simulink model "HIL_sim"  (Simulink 7.8)
settings: Solver=FixedStepDiscrete  StartTime=0.0  StopTime=1000  FixedStep=.01  RelTol=1e-3
InitFcn:
  | common
  | Busses
  | physical_constants
values from neighbouring files (symbols this model uses):
  T_step = 0.01    [boat_constants.m]    (also in common.m)
libraries: etargetslib x3, dspnetwork x2, simulink x1, aerolibanimutils x1
settings Model: Creator=Administrator  LastModifiedBy=Bryant  ExtModeAutoUpdateStatusClock=off  BufferReuse=off
settings DataIOCC: MaxDataPoints=1  SaveOutput=off  SignalLogging=off
settings OptimizationCC: BlockReduction=off  InlineParams=on  InlineInvariantSignals=on  BufferReuse=off  InitFltsAndDblsToZero=on  EfficientMapNaN2IntZero=off  LifeSpan=30  SimCompilerOptimization=On
settings DebuggingCC: ReadBeforeWriteMsg=DisableAll  SaveWithParameterizedLinksMsg=none  UnderspecifiedInitializationDetection=Simplified  UniqueDataStoreMsg=error  AssertControl=DisableAll
settings HardwareCC: ProdHWDeviceType=Generic->Unspecified (assume 32-bit Generic)  TargetIntDivRoundTo=Zero  TargetEndianess=LittleEndian  TargetHWDeviceType=Microchip->dsPIC
settings SFSimCC: SimParseCustomCode=off
settings CodeAppCC: MaxIdLength=128

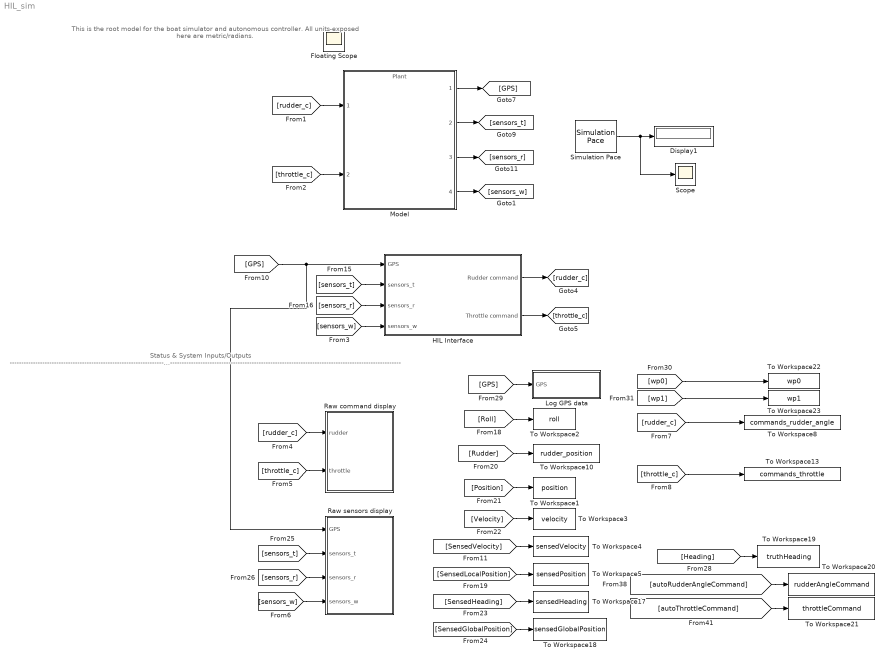
== system HIL_sim ==
  note: This is the root model for the boat simulator and autonomous controller. All
      | units exposed here are metric/radians.
  note: Status & System Inputs/Outputs
      | ---------------------------------------------------------------------------------------------------------------------------------------------------------------------------------------------------------------------------------------------------------
  Display1 : Display
      settings: Decimation=20
  HIL Interface : Subsystem
  Log GPS data : Subsystem
  Model : ModelReference  ModelNameDialog=Plant  SimulationMode=Normal  ModelReferenceVersion=1.14  CopyOfModelName=Plant  DefaultDataLogging=on
  Raw command display : Subsystem
  Raw sensors display : Subsystem
  Scope : Scope
      settings: SaveName=paceError  DataFormat=Array
  Simulation Pace : aerolibanimutils/Simulation Pace  SimulationPace=1  SleepMode=MATLAB Thread  OutputPaceError=on  SampleTime=T_step
      settings: AttributesFormatString=%<SimulationPace> sec/sec
  To Workspace1 : ToWorkspace  VariableName=position  SampleTime=-1  SaveFormat=Array
  To Workspace10 : ToWorkspace  VariableName=rudder_position  SampleTime=-1  SaveFormat=Array
  To Workspace13 : ToWorkspace  VariableName=commands_throttle  SampleTime=-1  SaveFormat=Array
  To Workspace17 : ToWorkspace  VariableName=sensedHeading  SampleTime=-1  SaveFormat=Array
  To Workspace18 : ToWorkspace  VariableName=sensedGlobalPosition  SampleTime=-1  SaveFormat=Array
  To Workspace19 : ToWorkspace  VariableName=truthHeading  SampleTime=-1  SaveFormat=Array
  To Workspace2 : ToWorkspace  VariableName=roll  SampleTime=-1  SaveFormat=Array
  To Workspace20 : ToWorkspace  VariableName=rudderAngleCommand  SampleTime=-1  SaveFormat=Array
  To Workspace21 : ToWorkspace  VariableName=throttleCommand  SampleTime=-1  SaveFormat=Array
  To Workspace22 : ToWorkspace  VariableName=wp0  SampleTime=-1  SaveFormat=Array
  To Workspace23 : ToWorkspace  VariableName=wp1  SampleTime=-1  SaveFormat=Array
  To Workspace3 : ToWorkspace  VariableName=velocity  SampleTime=-1  SaveFormat=Array
  To Workspace4 : ToWorkspace  VariableName=sensedVelocity  SampleTime=-1  SaveFormat=Array
  To Workspace5 : ToWorkspace  VariableName=sensedPosition  SampleTime=-1  SaveFormat=Array
  To Workspace8 : ToWorkspace  VariableName=commands_rudder_angle  SampleTime=-1  SaveFormat=Array
  Floating Scope : Scope
      settings: Floating=on
  wires:
  Model/3 -> [sensors_r]
  [rudder_c] -> Model/1
  [throttle_c] -> Model/2
  Model/1 -> [GPS]
  Model/2 -> [sensors_t]
  HIL Interface/1(Rudder command) -> [rudder_c]
  HIL Interface/2(Throttle command) -> [throttle_c]
  [sensors_r] -> HIL Interface/3(sensors_r)
  [sensors_t] -> HIL Interface/2(sensors_t)
  [GPS] -> HIL Interface/1(GPS), Raw sensors display/1(GPS)
  Model/4 -> [sensors_w]
  [rudder_c] -> Raw command display/1(rudder)
  [throttle_c] -> Raw command display/2(throttle)
  [sensors_t] -> Raw sensors display/2(sensors_t)
  [sensors_r] -> Raw sensors display/3(sensors_r)
  [Roll] -> To Workspace2/1
  [Rudder] -> To Workspace10/1
  [Position] -> To Workspace1/1
  [throttle_c] -> To Workspace13/1
  [rudder_c] -> To Workspace8/1
  [Velocity] -> To Workspace3/1
  [SensedVelocity] -> To Workspace4/1
  [SensedLocalPosition] -> To Workspace5/1
  [SensedHeading] -> To Workspace17/1
  [SensedGlobalPosition] -> To Workspace18/1
  [Heading] -> To Workspace19/1
  [autoRudderAngleCommand] -> To Workspace20/1
  [autoThrottleCommand] -> To Workspace21/1
  [GPS] -> Log GPS data/1(GPS)
  [wp0] -> To Workspace22/1
  [wp1] -> To Workspace23/1
  Simulation Pace/1 -> Display1/1, Scope/1
  [sensors_w] -> HIL Interface/4(sensors_w)
  [sensors_w] -> Raw sensors display/4(sensors_w)

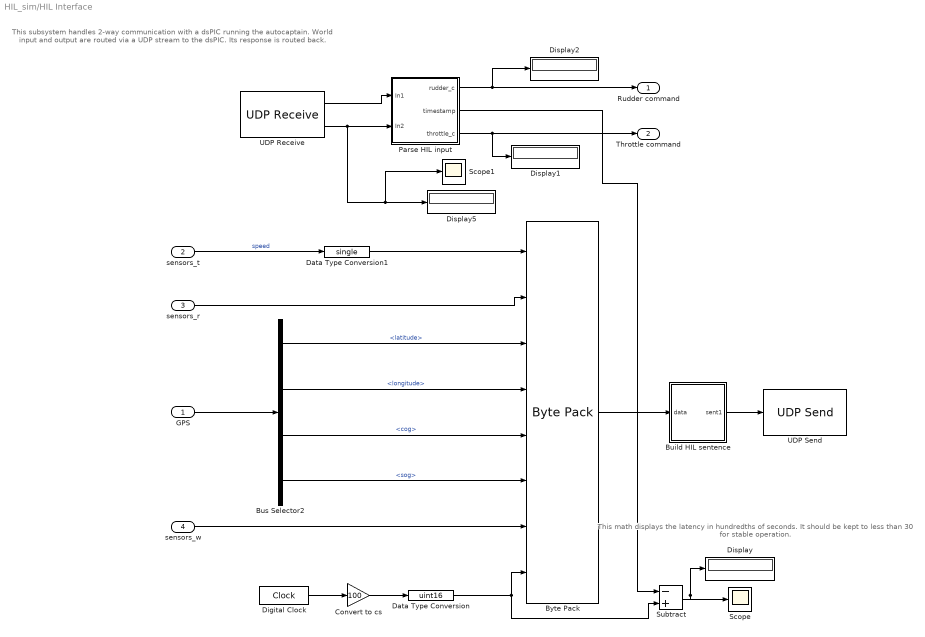
== system HIL_sim/HIL Interface ==
  note: This subsystem handles 2-way communication with a dsPIC running
      | the autocaptain. World input and output are routed via a UDP stream
      | to the dsPIC. Its response is routed back.
  note: This math displays the latency in hundredths of seconds.
      | It should be kept to less than 30 for stable operation.
  GPS : Inport
  sensors_t : Inport  Port=2
  sensors_r : Inport  Port=3
  sensors_w : Inport  Port=4
  Build HIL sentence : Subsystem
  Bus Selector2 : BusSelector  OutputSignals=latitude,longitude,cog,sog
  Byte Pack : etargetslib/Byte Pack  datatypes={'single','single','int32','int32','uint16','uint16','single','uint16'}  byteAlign=1
  Convert to cs : Gain  Gain=100
  Data Type Conversion : DataTypeConversion  OutDataTypeStr=uint16  RndMeth=Simplest
  Data Type Conversion1 : DataTypeConversion  OutDataTypeStr=single  RndMeth=Simplest
  Digital Clock : DigitalClock  SampleTime=.01
  Display{,1..2,5} (4 alike) : Display
  Parse HIL input : Subsystem
  Scope : Scope
      settings: YMin=40  YMax=92.5  SaveName=latency  DataFormat=Array
  Scope1 : Scope
      settings: YMin=40  YMax=92.5  SaveName=latency1  DataFormat=Array
  Subtract : Sum  Inputs=-+  OutDataTypeStr=int16
  UDP Receive : dspnetwork/UDP Receive  localURL='0.0.0.0'  localPort=14551  remoteURL='10.0.0.1'  remotePort=-1  recvBufferSize=44  dims=22  signalDatatype=uint8  isVarSize=off  showBlockingTime=on  blockingTime=0  sampletime=0.01  blockPlatform=HOST
  UDP Send : dspnetwork/UDP Send  remoteURL='10.0.0.1'  remotePort=14550  localURL='255.255.255.255'  localPortSource=Automatically determine  localPort=15000  sampletime=-1  blockPlatform=HOST  separateLengthPort=0
  Rudder command : Outport
  Throttle command : Outport  Port=2
  wires:
  Parse HIL input/1(rudder_c) -> Rudder command/1, Display2/1
  GPS/1 -> Bus Selector2/1
  Parse HIL input/3(throttle_c) -> Throttle command/1, Display1/1
  Byte Pack/1 -> Build HIL sentence/1(data)
  sensors_t/1 -> Data Type Conversion1/1  "speed"
  Build HIL sentence/1(sent1) -> UDP Send/1
  Parse HIL input/2(timestamp) -> Subtract/1
  Convert to cs/1 -> Data Type Conversion/1
  Digital Clock/1 -> Convert to cs/1
  Data Type Conversion/1 -> Subtract/2, Byte Pack/8
  Subtract/1 -> Scope/1, Display/1
  Data Type Conversion1/1 -> Byte Pack/1
  sensors_r/1 -> Byte Pack/2
  Bus Selector2/1 -> Byte Pack/3  "<latitude>"
  Bus Selector2/2 -> Byte Pack/4  "<longitude>"
  Bus Selector2/3 -> Byte Pack/5  "<cog>"
  Bus Selector2/4 -> Byte Pack/6  "<sog>"
  UDP Receive/1 -> Parse HIL input/1(In1)
  UDP Receive/2 -> Parse HIL input/2(In2), Display5/1, Scope1/1
  sensors_w/1 -> Byte Pack/7

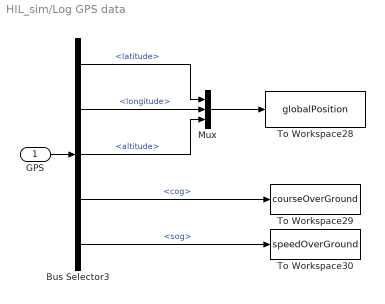
== system HIL_sim/Log GPS data ==
  GPS : Inport
  Bus Selector3 : BusSelector  OutputSignals=latitude,longitude,altitude,cog,sog
  Mux : Mux  Inputs=3
  To Workspace28 : ToWorkspace  VariableName=globalPosition  SampleTime=-1  SaveFormat=Array
  To Workspace29 : ToWorkspace  VariableName=courseOverGround  SampleTime=-1  SaveFormat=Array
  To Workspace30 : ToWorkspace  VariableName=speedOverGround  SampleTime=-1  SaveFormat=Array
  wires:
  Mux/1 -> To Workspace28/1
  Bus Selector3/1 -> Mux/1  "<latitude>"
  Bus Selector3/2 -> Mux/2  "<longitude>"
  Bus Selector3/3 -> Mux/3  "<altitude>"
  Bus Selector3/4 -> To Workspace29/1  "<cog>"
  Bus Selector3/5 -> To Workspace30/1  "<sog>"
  GPS/1 -> Bus Selector3/1

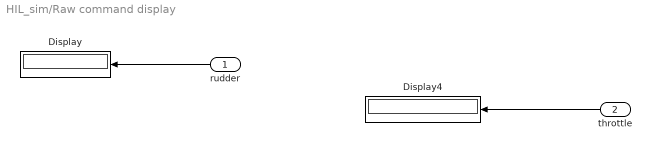
== system HIL_sim/Raw command display ==
  rudder : Inport
  throttle : Inport  Port=2
  Display : Display
  Display4 : Display
      settings: Format=hex (Stored Integer)
  wires:
  throttle/1 -> Display4/1
  rudder/1 -> Display/1

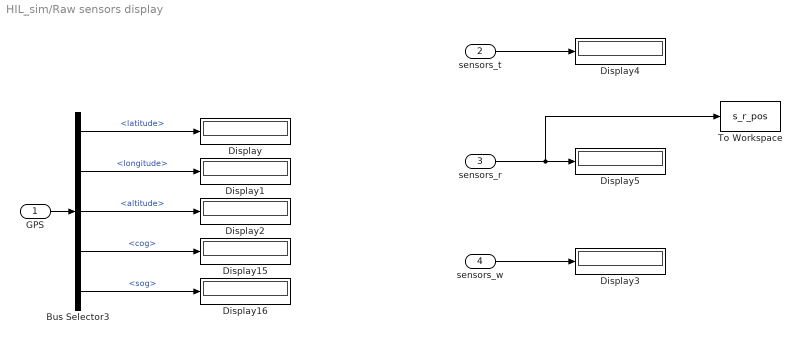
== system HIL_sim/Raw sensors display ==
  GPS : Inport
  sensors_t : Inport  Port=2
  sensors_r : Inport  Port=3
  sensors_w : Inport  Port=4
  Bus Selector3 : BusSelector  OutputSignals=latitude,longitude,altitude,cog,sog
  Display{,1..5,15..16} (8 alike) : Display
  To Workspace : ToWorkspace  VariableName=s_r_pos  SampleTime=-1  SaveFormat=Array
  wires:
  Bus Selector3/1 -> Display/1  "<latitude>"
  Bus Selector3/2 -> Display1/1  "<longitude>"
  Bus Selector3/3 -> Display2/1  "<altitude>"
  GPS/1 -> Bus Selector3/1
  sensors_t/1 -> Display4/1
  sensors_r/1 -> Display5/1, To Workspace/1
  Bus Selector3/4 -> Display15/1  "<cog>"
  Bus Selector3/5 -> Display16/1  "<sog>"
  sensors_w/1 -> Display3/1

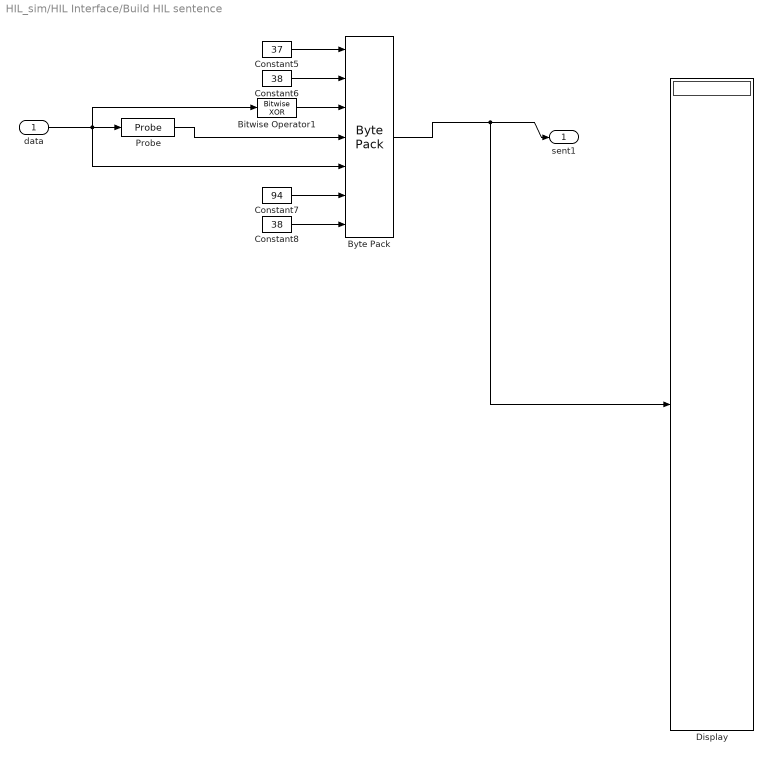
== system HIL_sim/HIL Interface/Build HIL sentence ==
  data : Inport
  Bitwise Operator1 : simulink/Logic and Bit Operations/Bitwise Operator  logicop=XOR  UseBitMask=off  BitMask=bin2dec('11011001')  BitMaskRealWorld=Stored Integer
  Byte Pack : etargetslib/Byte Pack  datatypes={'uint8', 'uint8', 'uint8', 'uint8', 'uint8', 'uint8', 'uint8'}  byteAlign=1
  Constant5 : Constant  Value=37  OutDataTypeStr=uint8
  Constant6 : Constant  Value=38  OutDataTypeStr=uint8
  Constant7 : Constant  Value=94  OutDataTypeStr=uint8
  Constant8 : Constant  Value=38  OutDataTypeStr=uint8
  Display : Display
  Probe : Probe  ProbeSampleTime=off  ProbeComplexSignal=off  ProbeWidthDataType=uint8
  sent1 : Outport
  wires:
  Constant5/1 -> Byte Pack/1
  Constant6/1 -> Byte Pack/2
  Probe/1 -> Byte Pack/4
  Constant7/1 -> Byte Pack/6
  Constant8/1 -> Byte Pack/7
  Bitwise Operator1/1 -> Byte Pack/3
  data/1 -> Probe/1, Byte Pack/5, Bitwise Operator1/1
  Byte Pack/1 -> sent1/1, Display/1

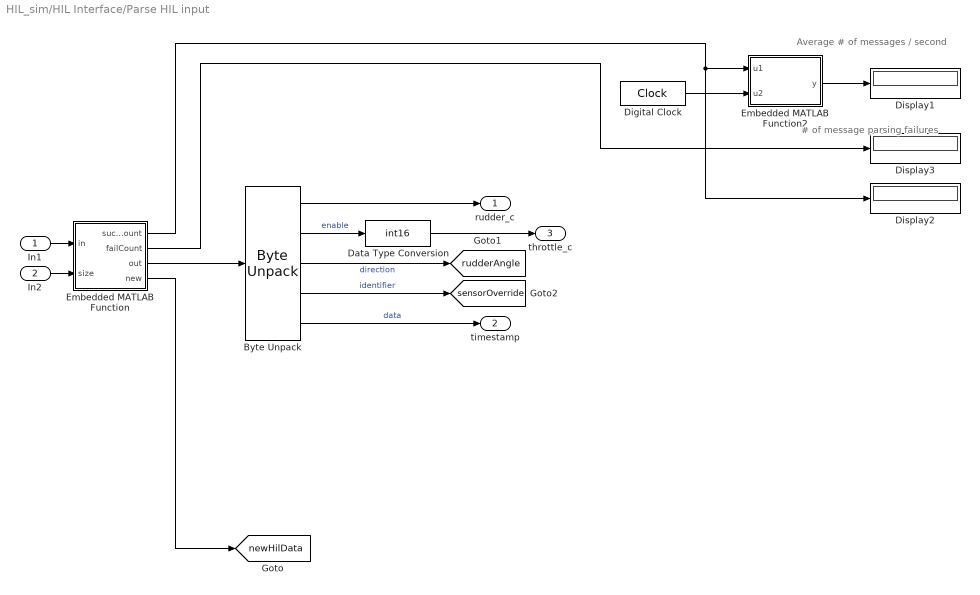
== system HIL_sim/HIL Interface/Parse HIL input ==
  note: # of message parsing failures
  note: Average # of messages / second
  In1 : Inport
  In2 : Inport  Port=2
  Byte Unpack : etargetslib/Byte Unpack  dimensions={1, 1, 1, 1, 1}  datatypes={'single', 'single', 'single', 'uint16', 'uint16'}  byteAlign=1
  Data Type Conversion : DataTypeConversion  OutDataTypeStr=int16  RndMeth=Simplest
  Digital Clock : DigitalClock  SampleTime=T_step
  Display1 : Display
  Display2 : Display
  Display3 : Display
  Embedded MATLAB Function : MATLAB Function  TreatAsAtomicUnit=on
  Embedded MATLAB Function2 : MATLAB Function  TreatAsAtomicUnit=on
  rudder_c : Outport
  timestamp : Outport  Port=2
  throttle_c : Outport  Port=3
  tag scope: newHilData=global, rudderAngle=global, sensorOverride=global
  wires:
  Embedded MATLAB Function/3(out) -> Byte Unpack/1
  In1/1 -> Embedded MATLAB Function/1(in)
  Embedded MATLAB Function/1(successCount) -> Embedded MATLAB Function2/1(u1), Display2/1
  Digital Clock/1 -> Embedded MATLAB Function2/2(u2)
  Embedded MATLAB Function2/1(y) -> Display1/1
  Embedded MATLAB Function/2(failCount) -> Display3/1
  Byte Unpack/4 -> [sensorOverride]  "identifier"
  Embedded MATLAB Function/4(new) -> [newHilData]
  Byte Unpack/5 -> timestamp/1  "data"
  Byte Unpack/1 -> rudder_c/1
  Byte Unpack/2 -> Data Type Conversion/1  "enable"
  Byte Unpack/3 -> [rudderAngle]  "direction"
  In2/1 -> Embedded MATLAB Function/2(size)
  Data Type Conversion/1 -> throttle_c/1

== matlab function HIL Interface/Parse HIL input/Embedded MATLAB Function ==
  data: successCount output double; failCount output double; in input uint8; out output uint8 size=16; new output double; size input double
function [successCount, failCount, out, new] = parseMessage(in, size)
    persistent actuatorMessage internalSuccessCount internalFailCount;
    
    if isempty(actuatorMessage)
        actuatorMessage = zeros(16, 1, 'uint8');
        internalSuccessCount = uint32(0);
        internalFailCount = uint32(0);
    end
    
    newData = false;
    for k = 1:size
        [newData fail data] = buildAndCheckMessage(in(k));
        if newData
            actuatorMessage = data;
            internalSuccessCount = internalSuccessCount + 1;
        elseif fail
            internalFailCount = internalFailCount + 1;
        end
    end
    successCount = internalSuccessCount;
    failCount = internalFailCount;
    out = actuatorMessage;
    new = newData;
end

function [new fail data] = buildAndCheckMessage(characterIn)

    persistent message messageIndex messageState actuatorData;

    if isempty(message)
        message = zeros(22, 1, 'uint8');
        messageIndex = uint8(0);
        messageState = uint8(0);
        actuatorData = zeros(16, 1, 'uint8');
    end

    % This contains the function's state of whether
    % it is currently building a message.
    % 0 - Awaiting header byte 0 (%)
    % 1 - Awaiting header byte 1 (&)
    % 2 - Building message
    % 3 - Awaiting header byte 0 (^)
    % 4 - Awaiting header byte 1 (&)
    % 5 - Reading checksum character

    new = false;
    fail = false;

    % We start recording a new message if we see the header
    if messageState == 0
        if characterIn == '%'
            messageIndex = uint8(1);
            message(messageIndex) = characterIn;
            messageIndex = messageIndex + 1;
            messageState = uint8(1);
        else
            fail = true;
        end
    elseif messageState == 1
        % If we don't find the necessary ampersand we start over
        % waiting for a new sentence
        if characterIn == '&'
            message(messageIndex) = characterIn;
            messageIndex = messageIndex + 1;
            messageState = uint8(2);
        elseif characterIn ~= '%'
            messageIndex = uint8(1);
            messageState = uint8(0);
            fail = true;
        end
    elseif messageState == 2
        % Record every character that comes in now that we're building a sentence.
        % Only stop if we run out of room or an asterisk is found.
        message(messageIndex) = characterIn;
        messageIndex = messageIndex + 1;
        if messageIndex > 4 && message(4) < 249 && messageIndex == message(4) + 6
            if characterIn == '^'
                messageState = uint8(3);
            else
                messageIndex = uint8(1);
                messageState = uint8(0);
                fail = true;
            end
        elseif messageIndex == length(message)
            % If we've filled up the buffer, ignore the entire message as we can't store it all
            messageIndex = uint8(1);
            messageState = uint8(0);
            fail = true;
        end
    elseif messageState == 3
        message(messageIndex) = characterIn;
        % If we don't find the necessary ampersand we continue
        % recording data as we haven't found the footer yet until
        % we've filled up the entire message (ends at 124 characters
        % as we need room for the 2 footer chars).
        if characterIn == '&'

            % The checksum is now verified and if successful the message
            % is stored in the appropriate struct.
            checksumCalculated = uint8(0);
            for f=5:messageIndex-2
                checksumCalculated = bitxor(checksumCalculated, message(f));
            end

            if message(3) == checksumCalculated
                % If we've found an actuator message, update our local data store
                actuatorData = message(5:5+length(actuatorData)-1);
                new = true;
            else
                fail = true;
            end
        end

        % We clear all state variables here regardless of success.
        messageIndex = uint8(1);
        messageState = uint8(0);
        message = zeros(22,1,'uint8');
    end

    data = actuatorData;
end

== matlab function HIL Interface/Parse HIL input/Embedded MATLAB Function2 ==
  data: u1 input double; y output double; u2 input double
function y = safeDiv(u1, u2)
%#eml

if u2 == 0
    y = u1;
else
    y = u1 / u2;
end
